simulink model "AW_comp"  (R2019b)
settings: Solver=ode5  StartTime=0.0  StopTime=200  FixedStep=0.001  RelTol=1e-3
values from neighbouring files (symbols this model uses):
  G = ss(4/(s^2+0.1*s+1))    [Demo_003.m]    (also in Demo_009.m = tf(1,[k^2,2*d*k,1]); Demo_010.m = ss(10/(100*s+1)*[4,-5;-3,4]); Demo_011.m = rss(n,1,2); Demo_012.m = Gnom*(1+W*Delta))
  K = ss(zeros(2),eye(2),[2,2.5;1.5,2]/100,[2,2.5;1.5,2])    [Demo_010.m]    (also in Demo_013.m = null(Wi-C'/H*C); Demo_015.m = ss(aK,bK,cK,dK)*diag(diag(Jnom)))
  Ke = ss(K.a,[K.b,eye(2),zeros(2)],K.c,[K.d,zeros(2),eye(2)])    [Demo_010.m]
undefined symbols (not defined in the file or in its folder): Kaw
settings Model: Creator=joost.veenman  LastModifiedBy=joost.veenman

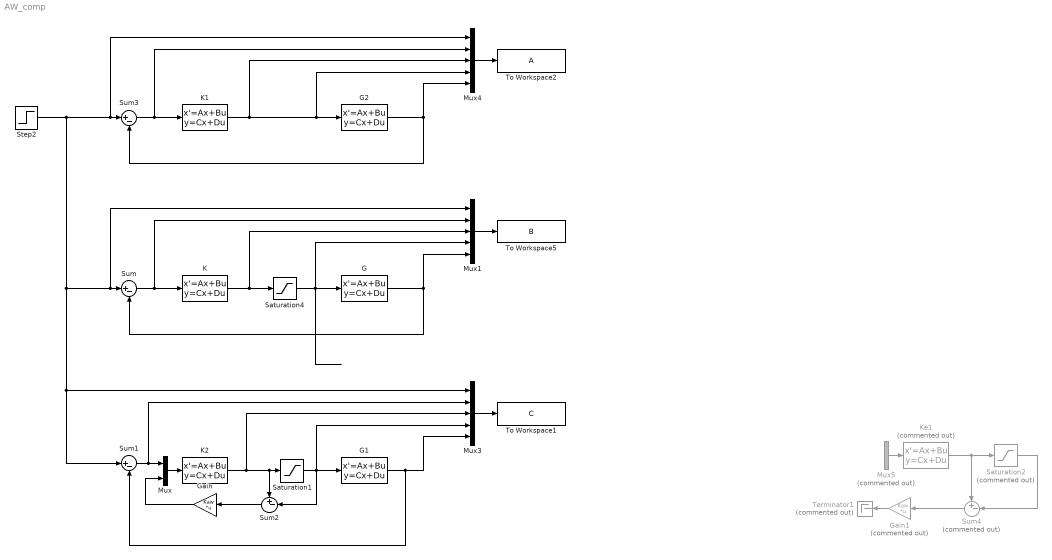
== system AW_comp ==
  G : StateSpace  A=G.a  B=G.b  C=G.c  D=G.d  InitialCondition=0
  G1 : StateSpace  A=G.a  B=G.b  C=G.c  D=G.d  InitialCondition=0
  G2 : StateSpace  A=G.a  B=G.b  C=G.c  D=G.d  InitialCondition=0
  Gain : Gain  Gain=Kaw  Multiplication=Matrix(K*u)
  Gain1 : Gain  Commented=on  Gain=Kaw  Multiplication=Matrix(K*u)
  K : StateSpace  A=K.a  B=K.b  C=K.c  D=K.d  InitialCondition=0
  K1 : StateSpace  A=K.a  B=K.b  C=K.c  D=K.d  InitialCondition=0
  K2 : StateSpace  A=Ke.a  B=Ke.b  C=Ke.c  D=Ke.d  InitialCondition=0
  Ke1 : StateSpace  Commented=on  A=Ke.a  B=Ke.b  C=Ke.c  D=Ke.d  InitialCondition=0
  Mux : Mux  Inputs=2
  Mux1 : Mux  Inputs=5
  Mux3 : Mux  Inputs=5
  Mux4 : Mux  Inputs=5
  Mux5 : Mux  Commented=on  Inputs=2
  Saturation1 : Saturate  UpperLimit=1  LowerLimit=-1
  Saturation2 : Saturate  Commented=on  UpperLimit=1  LowerLimit=-1
  Saturation4 : Saturate  UpperLimit=1  LowerLimit=-1
  Step2 : Step  Time=0  After=[0.63;0.79]  SampleTime=0
  Sum : Sum  Inputs=|+-
  Sum1 : Sum  Inputs=|+-
  Sum2 : Sum  Inputs=+-|
  Sum3 : Sum  Inputs=|+-
  Sum4 : Sum  Commented=on  Inputs=+-|
  Terminator1 : Terminator  Commented=on
  To Workspace1 : ToWorkspace  VariableName=C  SaveFormat=Timeseries  SampleTime=-1
  To Workspace2 : ToWorkspace  VariableName=A  SaveFormat=Timeseries  SampleTime=-1
  To Workspace5 : ToWorkspace  VariableName=B  SaveFormat=Timeseries  SampleTime=-1
  wires:
  Saturation4/1 -> G/1, Mux1/4
  K/1 -> Mux1/3, Saturation4/1
  Sum/1 -> Mux1/2, K/1
  G/1 -> Mux1/5, Sum/2
  Mux1/1 -> To Workspace5/1
  Mux3/1 -> To Workspace1/1
  Saturation1/1 -> Sum2/2, Mux3/4, G1/1
  Sum1/1 -> Mux/1, Mux3/2
  G1/1 -> Mux3/5, Sum1/2
  Mux4/1 -> To Workspace2/1
  K1/1 -> Mux4/4, G2/1, Mux4/3
  Sum3/1 -> Mux4/2, K1/1
  Step2/1 -> Mux4/1, Sum3/1, Mux1/1, Sum/1, Mux3/1, Sum1/1
  G2/1 -> Mux4/5, Sum3/2
  Sum4/1 -> Gain1/1
  Ke1/1 -> Sum4/1, Saturation2/1
  Mux5/1 -> Ke1/1
  Saturation2/1 -> Sum4/2
  Gain1/1 -> Terminator1/1
  K2/1 -> Mux3/3, Sum2/1, Saturation1/1
  Gain/1 -> Mux/2
  Mux/1 -> K2/1
  Sum2/1 -> Gain/1
